simulink model "PV_hacheur_PJT_MODIFIE"  (R2017b)
settings: Solver=ode1  StartTime=0.0  StopTime=t_simul  FixedStep=pas_calcul  RelTol=1e-3  EnableMultiTasking=on
values from neighbouring files (symbols this model uses):
  a = 1.2    [init_hacheur_PV_MODIFIE.m]
  DeltaI = 0.1    [init_hacheur_PV_MODIFIE.m]
  E = 1500    [init_hacheur_PV_MODIFIE.m]
  Gstc = 1000    [init_hacheur_PV_MODIFIE.m]
  Isc = 3.8    [init_hacheur_PV_MODIFIE.m]
  K = 1.38*10^(-23)    (= 1.38e-23)    [init_hacheur_PV_MODIFIE.m]
  Kisc = 0.024    [init_hacheur_PV_MODIFIE.m]
  Kvco = -0.08    [init_hacheur_PV_MODIFIE.m]
  L = Lmin    (= 0.012)    [init_hacheur_PV_MODIFIE.m]
  Ns = 36    [init_hacheur_PV_MODIFIE.m]
  pas_calcul = 1e-6    (= 1e-06)    [init_hacheur_PV_MODIFIE.m]
  q = 1.6*10^(-19)    (= 1.6e-19)    [init_hacheur_PV_MODIFIE.m]
  Rl = L    (= 0.012)    [init_hacheur_PV_MODIFIE.m]
  Rs = 0.008    [init_hacheur_PV_MODIFIE.m]
  Rsh = 1000    [init_hacheur_PV_MODIFIE.m]
  t_simul = 0.1    [init_hacheur_PV_MODIFIE.m]
  Tc = 15+273    (= 288)    [init_hacheur_PV_MODIFIE.m]
  Tstc = 25+273    (= 298)    [init_hacheur_PV_MODIFIE.m]
  Vco = 21.1    [init_hacheur_PV_MODIFIE.m]
  Vdc = 60    [init_hacheur_PV_MODIFIE.m]
  VpvREF = 19    [init_hacheur_PV_MODIFIE.m]
libraries: powerlib x10, simulink_extras x1
settings Model: Creator=adm-gruson  LastModifiedBy=hl9499
settings SolverCC: AutoInsertRateTranBlk=on
settings DataIOCC: LimitDataPoints=on  SaveFormat=Array
settings OptimizationCC: LifeSpan=inf
settings DebuggingCC: SFUnexpectedBacktrackingDiag=warning  SFNoUnconditionalDefaultTransitionDiag=warning  SFExecutionAtInitializationDiag=none
settings HardwareCC: ProdBitPerPointer=32  ProdBitPerSizeT=32  ProdBitPerPtrDiffT=32  ProdLargestAtomicFloat=None  ProdIntDivRoundTo=Undefined  ProdEndianess=Unspecified  ProdWordSize=32  ProdHWDeviceType=32-bit Generic
settings ModelReferenceCC: PropagateSignalLabelsOutOfModel=off
settings CodeAppCC: StateflowObjectComments=on
settings GRTTargetCC: TargetLangStandard=C89/C90 (ANSI)  GeneratePreprocessorConditionals=Disable all
settings ConfigComp: CovMetricSettings=dw  CovHtmlReporting=on  CovSaveCumulativeToWorkspaceVar=on  CovSaveSingleToWorkspaceVar=on  CovExternalEMLEnable=off
settings SimscapeCC: SimscapeNormalizeSystem=off

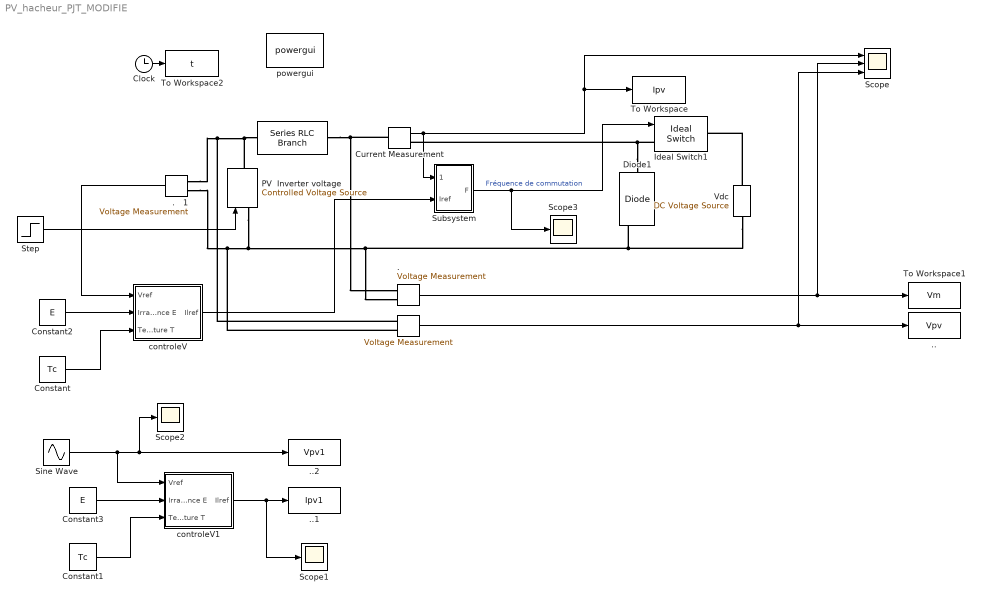
== system PV_hacheur_PJT_MODIFIE ==
  "  " : powerlib/Elements/Series RLC Branch  LConnTagsString=__new0  RConnTagsString=__new0  BranchType=RL  Resistance=L  Inductance=Rl  SetiL0=off  InitialCurrent=0  Capacitance=1e-6  Setx0=off  InitialVoltage=0  Measurements=None
  "      " : powerlib/Measurements/Voltage Measurement  PhasorSimulation=off  OutputType=Complex  PSBequivalent=0
  ".   " : powerlib/Measurements/Voltage Measurement  PhasorSimulation=off  OutputType=Complex  PSBequivalent=0
  .   1 : powerlib/Measurements/Voltage Measurement  PhasorSimulation=off  OutputType=Complex  PSBequivalent=0
  .. : ToWorkspace  VariableName=Vpv  SampleTime=-1
  ..1 : ToWorkspace  VariableName=Ipv1  SampleTime=-1
  ..2 : ToWorkspace  VariableName=Vpv1  SampleTime=-1
  Clock : Clock
  Constant : Constant  Value=Tc  SampleTime=-1
  Constant1 : Constant  Value=Tc  SampleTime=-1
  Constant2 : Constant  Value=E  SampleTime=-1
  Constant3 : Constant  Value=E  SampleTime=-1
  Current Measurement : powerlib/Measurements/Current Measurement  PhasorSimulation=off  OutputType=Complex  PSBequivalent=0
  Diode1 : powerlib/Power Electronics/Diode  Ron=0.001  Lon=0  Vf=0  IC=0  UseSnubber=off  Rs=500000  Cs=250e-6  Measurements=on
  Ideal Switch1 : powerlib/Power Electronics/Ideal Switch  Ron=0.001  Lon=0  IC=0  Rs=1e5  Cs=inf  Measurements=off
  PV  Inverter voltage : powerlib/Electrical Sources/Controlled Voltage Source  Initialize=on  Source_Type=DC  Amplitude=VpvREF  Phase=0  Frequency=0  Measurements=None
  Scope : Scope  NumInputPorts=3
  Scope1 : Scope
  Scope2 : Scope
  Scope3 : Scope
  Sine Wave : Sin  Amplitude=-VpvREF-10  Frequency=1/t_simul  Phase=-pi  SampleTime=0
  Step : Step  Time=0.05  Before=VpvREF  After=0.9*VpvREF  SampleTime=0
  Subsystem : Subsystem
  To Workspace : ToWorkspace  VariableName=Ipv  SampleTime=-1
  To Workspace1 : ToWorkspace  VariableName=Vm  SampleTime=-1
  To Workspace2 : ToWorkspace  VariableName=t  SampleTime=-1
  Vdc : powerlib/Electrical Sources/DC Voltage Source  Amplitude=Vdc  Measurements=None
  controleV : Subsystem
  controleV1 : Subsystem
  powergui : powerlib/powergui  Priority=1  SimulationMode=Discrete  SampleTime=pas_calcul  frequency=60  Iterations=50  frequencyindice=0  Pbase=100e6  ErrMax=1e-4  UnitsV=kV  UnitsW=MW  buscounter=0  FunctionMessages=off  echomessages=off  EnableUseOfTLC=off  CurrentSourceSwitches=off  DisableSnubberDevices=off  DisableRonSwitches=off  DisableVfSwitches=off  DisplayEquations=off  SolverType=Tustin/Backward Euler (TBE)  Interpol=off  ExternalGateDelay=off  methode=off  Ts=100  x0status=blocks  SPID=off  SwTol=0  HookPort=off  RestoreLinks=warning  ResistiveCurrentMeasurement=off  Frange=[0:2:500]  Ylog=off  Xlog=on  ShowGrid=off  save=off  variable=ZData  structure=0  ZoomFFT=off  StartTime=0.0  cycles=1  DisplayStyle=1  fundamental=60  FreqAxis=off  MaxFrequency=1000  frequencyindicesteady=1  RmsSteady=1  display=off
  wires:
  Current Measurement/1 -> Subsystem/1(Imes), To Workspace/1, Scope/1
  Clock/1 -> To Workspace2/1
  ".   "/1 -> Scope/2, To Workspace1/1
  "      "/1 -> Scope/3, ../1
  controleV/1(Ilref) -> Subsystem/2(Iref)
  Constant2/1 -> controleV/2(Irradiance E)
  Constant/1 -> controleV/3(Temperature T)
  Subsystem/1(F) -> Scope3/1, Ideal Switch1/1  "Fréquence de commutation"
  .   1/1 -> controleV/1("Vref ")
  Step/1 -> PV  Inverter voltage/1
  Constant1/1 -> controleV1/3(Temperature T)
  Constant3/1 -> controleV1/2(Irradiance E)
  controleV1/1(Ilref) -> Scope1/1, ..1/1
  Sine Wave/1 -> controleV1/1("Vref "), Scope2/1, ..2/1
  connections:
  Current Measurement/LConn1 -- "  "/RConn1 -- ".   "/LConn1
  Vdc/LConn1 -- Diode1/RConn1 -- .   1/LConn2 -- "      "/LConn2 -- PV  Inverter voltage/LConn1 -- ".   "/LConn2
  Diode1/LConn1 -- Current Measurement/RConn1 -- Ideal Switch1/LConn1
  Vdc/RConn1 -- Ideal Switch1/RConn1
  PV  Inverter voltage/RConn1 -- "      "/LConn1 -- .   1/LConn1 -- "  "/LConn1

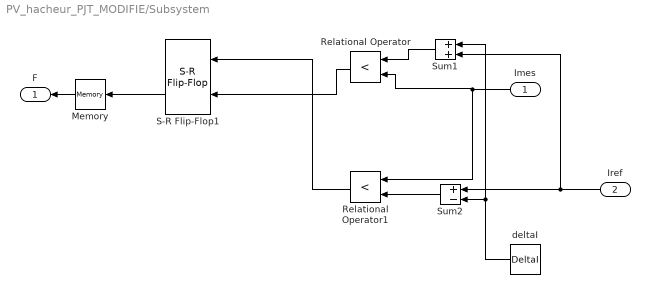
== system PV_hacheur_PJT_MODIFIE/Subsystem ==
  Imes : Inport
  Iref : Inport  Port=2
  Memory : Memory  InheritSampleTime=on
  Relational Operator : RelationalOperator  Operator=<  OutDataTypeStr=boolean  RndMeth=Nearest
  Relational Operator1 : RelationalOperator  Operator=<  OutDataTypeStr=boolean  RndMeth=Nearest
  S-R Flip-Flop1 : simulink_extras/Flip Flops/S-R Flip-Flop  initial_condition=0
  Sum1 : Sum
  Sum2 : Sum  Inputs=+-
  deltaI : Constant  Value=DeltaI
  F : Outport
  wires:
  Memory/1 -> F/1
  Relational Operator/1 -> S-R Flip-Flop1/2
  Relational Operator1/1 -> S-R Flip-Flop1/1
  Imes/1 -> Relational Operator/2, Relational Operator1/1
  Sum2/1 -> Relational Operator1/2
  deltaI/1 -> Sum2/2, Sum1/1
  Sum1/1 -> Relational Operator/1
  Iref/1 -> Sum1/2, Sum2/1
  S-R Flip-Flop1/2 -> Memory/1

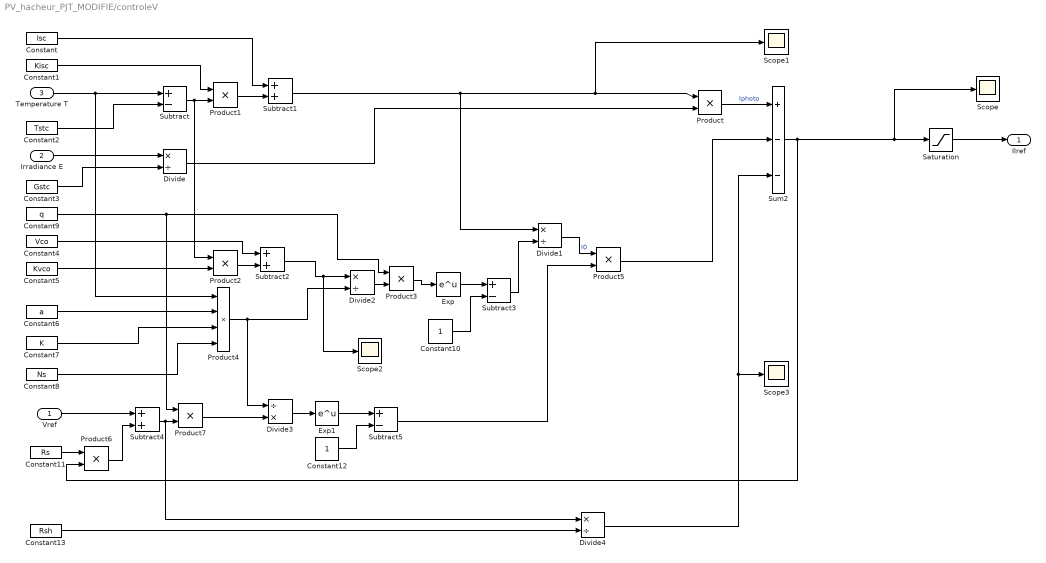
== system PV_hacheur_PJT_MODIFIE/controleV ==
  "Vref " : Inport
  Irradiance E : Inport  Port=2
  Temperature T : Inport  Port=3
  Constant : Constant  Value=Isc  SampleTime=-1
  Constant1 : Constant  Value=Kisc  SampleTime=-1
  Constant10 : Constant  SampleTime=-1
  Constant11 : Constant  Value=Rs  SampleTime=-1
  Constant12 : Constant  SampleTime=-1
  Constant13 : Constant  Value=Rsh  SampleTime=-1
  Constant2 : Constant  Value=Tstc  SampleTime=-1
  Constant3 : Constant  Value=Gstc  SampleTime=-1
  Constant4 : Constant  Value=Vco  SampleTime=-1
  Constant5 : Constant  Value=Kvco  SampleTime=-1
  Constant6 : Constant  Value=a  SampleTime=-1
  Constant7 : Constant  Value=K  SampleTime=-1
  Constant8 : Constant  Value=Ns  SampleTime=-1
  Constant9 : Constant  Value=q  SampleTime=-1
  Divide{,1..2,4} (4 alike) : Product  Inputs=*/
  Divide3 : Product  Inputs=/*
  Exp : Math  SaturateOnIntegerOverflow=on
  Exp1 : Math  SaturateOnIntegerOverflow=on
  Product{,1..3,5..7} (7 alike) : Product
  Product4 : Product  Inputs=4
  Saturation : Saturate  UpperLimit=150  LowerLimit=0
  Scope{,1..3} (4 alike) : Scope
  Subtract : Sum  Inputs=+-
  Subtract1 : Sum
  Subtract2 : Sum
  Subtract3 : Sum  Inputs=+-
  Subtract4 : Sum
  Subtract5 : Sum  Inputs=+-
  Sum2 : Sum  Inputs=+--  SaturateOnIntegerOverflow=on  InputSameDT=on  OutDataTypeStr=Inherit: Same as first input
  Ilref : Outport
  wires:
  Irradiance E/1 -> Divide/1
  Constant3/1 -> Divide/2
  Divide/1 -> Product/2
  Temperature T/1 -> Product4/1, Subtract/1
  Constant2/1 -> Subtract/2
  Subtract/1 -> Product1/2, Product2/1
  Constant1/1 -> Product1/1
  Product1/1 -> Subtract1/2
  Constant/1 -> Subtract1/1
  Subtract1/1 -> Divide1/1, Scope1/1, Product/1
  Product/1 -> Sum2/1  "Iphoto"
  Constant5/1 -> Product2/2
  Product2/1 -> Subtract2/2
  Constant4/1 -> Subtract2/1
  Constant9/1 -> Product7/1, Product3/1
  Subtract2/1 -> Scope2/1, Divide2/1
  Constant6/1 -> Product4/2
  Constant7/1 -> Product4/3
  Constant8/1 -> Product4/4
  Product4/1 -> Divide3/1, Divide2/2
  Exp/1 -> Subtract3/1
  Constant10/1 -> Subtract3/2
  Subtract3/1 -> Divide1/2
  Divide1/1 -> Product5/1  "I0"
  Constant11/1 -> Product6/1
  Product6/1 -> Subtract4/2
  Subtract4/1 -> Divide4/1, Product7/2
  Product7/1 -> Divide3/2
  Divide3/1 -> Exp1/1
  Exp1/1 -> Subtract5/1
  Constant12/1 -> Subtract5/2
  Subtract5/1 -> Product5/2
  Product5/1 -> Sum2/2
  Constant13/1 -> Divide4/2
  Divide4/1 -> Scope3/1, Sum2/3
  Sum2/1 -> Product6/2, Scope/1, Saturation/1
  Divide2/1 -> Product3/2
  Product3/1 -> Exp/1
  "Vref "/1 -> Subtract4/1
  Saturation/1 -> Ilref/1

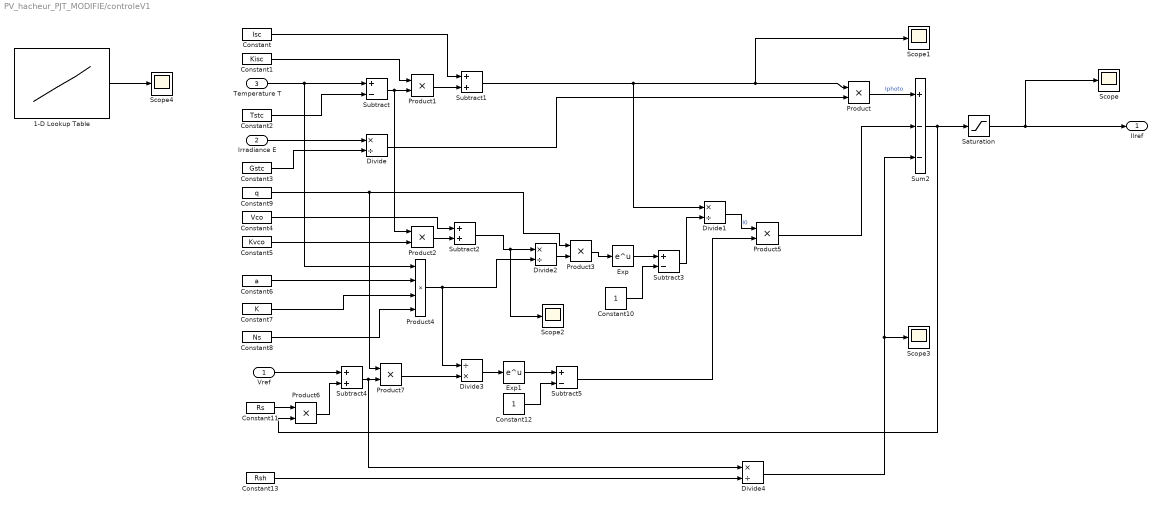
== system PV_hacheur_PJT_MODIFIE/controleV1 ==
  "Vref " : Inport
  Irradiance E : Inport  Port=2
  Temperature T : Inport  Port=3
  1-D Lookup Table : Lookup_n-D  NumberOfTableDimensions=1  BreakpointsForDimension1=[0,0.0024,0.0048,0.0072,0.0096,0.012,0.0144,0.0168,0.0192,0.0216,0.024,0.0264,0.0288,0.0312,0.0336,0.036,0.0384,0.0406,0.0432,0.0456,0.048,0.0504,0.0528,0.0552,0.0576,0.06,0.0624,0.0648,0.0672,0.0696,0.072,0.0744,0.0768,0.0792,0.0816,0.084,0.0864,0.0888,0.0912,0.0936,0.096,0.1]  Table=[0,0.5,1,1.5,2,2.5,3,3.5,4,4.5,5,5.5,6,6.5,7,7.5,8,8.5,9,9.5,10,10.5,11,11.5,12,12.5,13,13.5,14,14.5,15,15.5,16,16.5,17,17.5,18,18.5,19,19.5,20,20.5]  InternalRulePriority=Speed  RndMeth=Simplest  InputSameDT=on
  Constant : Constant  Value=Isc  SampleTime=-1
  Constant1 : Constant  Value=Kisc  SampleTime=-1
  Constant10 : Constant  SampleTime=-1
  Constant11 : Constant  Value=Rs  SampleTime=-1
  Constant12 : Constant  SampleTime=-1
  Constant13 : Constant  Value=Rsh  SampleTime=-1
  Constant2 : Constant  Value=Tstc  SampleTime=-1
  Constant3 : Constant  Value=Gstc  SampleTime=-1
  Constant4 : Constant  Value=Vco  SampleTime=-1
  Constant5 : Constant  Value=Kvco  SampleTime=-1
  Constant6 : Constant  Value=a  SampleTime=-1
  Constant7 : Constant  Value=K  SampleTime=-1
  Constant8 : Constant  Value=Ns  SampleTime=-1
  Constant9 : Constant  Value=q  SampleTime=-1
  Divide{,1..2,4} (4 alike) : Product  Inputs=*/
  Divide3 : Product  Inputs=/*
  Exp : Math  SaturateOnIntegerOverflow=on
  Exp1 : Math  SaturateOnIntegerOverflow=on
  Product{,1..3,5..7} (7 alike) : Product
  Product4 : Product  Inputs=4
  Saturation : Saturate  UpperLimit=150  LowerLimit=0
  Scope{,1..4} (5 alike) : Scope
  Subtract : Sum  Inputs=+-
  Subtract1 : Sum
  Subtract2 : Sum
  Subtract3 : Sum  Inputs=+-
  Subtract4 : Sum
  Subtract5 : Sum  Inputs=+-
  Sum2 : Sum  Inputs=+--  SaturateOnIntegerOverflow=on  InputSameDT=on  OutDataTypeStr=Inherit: Same as first input
  Ilref : Outport
  wires:
  "Vref "/1 -> Subtract4/1
  1-D Lookup Table/1 -> Scope4/1
  Product3/1 -> Exp/1
  Divide2/1 -> Product3/2
  Sum2/1 -> Saturation/1, Product6/2
  Divide4/1 -> Sum2/3, Scope3/1
  Constant13/1 -> Divide4/2
  Product5/1 -> Sum2/2
  Subtract5/1 -> Product5/2
  Constant12/1 -> Subtract5/2
  Exp1/1 -> Subtract5/1
  Divide3/1 -> Exp1/1
  Product7/1 -> Divide3/2
  Subtract4/1 -> Product7/2, Divide4/1
  Product6/1 -> Subtract4/2
  Constant11/1 -> Product6/1
  Divide1/1 -> Product5/1  "I0"
  Subtract3/1 -> Divide1/2
  Constant10/1 -> Subtract3/2
  Exp/1 -> Subtract3/1
  Product4/1 -> Divide2/2, Divide3/1
  Constant8/1 -> Product4/4
  Constant7/1 -> Product4/3
  Constant6/1 -> Product4/2
  Subtract2/1 -> Divide2/1, Scope2/1
  Constant9/1 -> Product3/1, Product7/1
  Constant4/1 -> Subtract2/1
  Product2/1 -> Subtract2/2
  Constant5/1 -> Product2/2
  Product/1 -> Sum2/1  "Iphoto"
  Subtract1/1 -> Product/1, Scope1/1, Divide1/1
  Constant/1 -> Subtract1/1
  Product1/1 -> Subtract1/2
  Constant1/1 -> Product1/1
  Subtract/1 -> Product2/1, Product1/2
  Constant2/1 -> Subtract/2
  Temperature T/1 -> Subtract/1, Product4/1
  Divide/1 -> Product/2
  Constant3/1 -> Divide/2
  Irradiance E/1 -> Divide/1
  Saturation/1 -> Ilref/1, Scope/1
